simulink model "sampleModel2087"  (R2023a)
settings: Solver=VariableStepAuto  StartTime=0.0  StopTime=10.0  RelTol=1e-3
libraries: simulink x4, hdlsllib x3
settings Model: Creator=user1  LastModifiedBy=user1

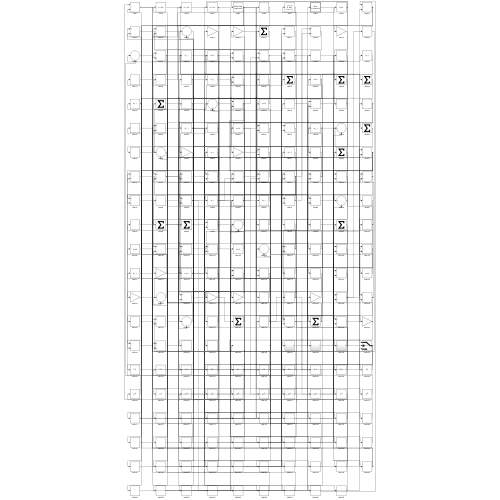
[thumbnail: Simulink's stored preview of the top-level diagram]
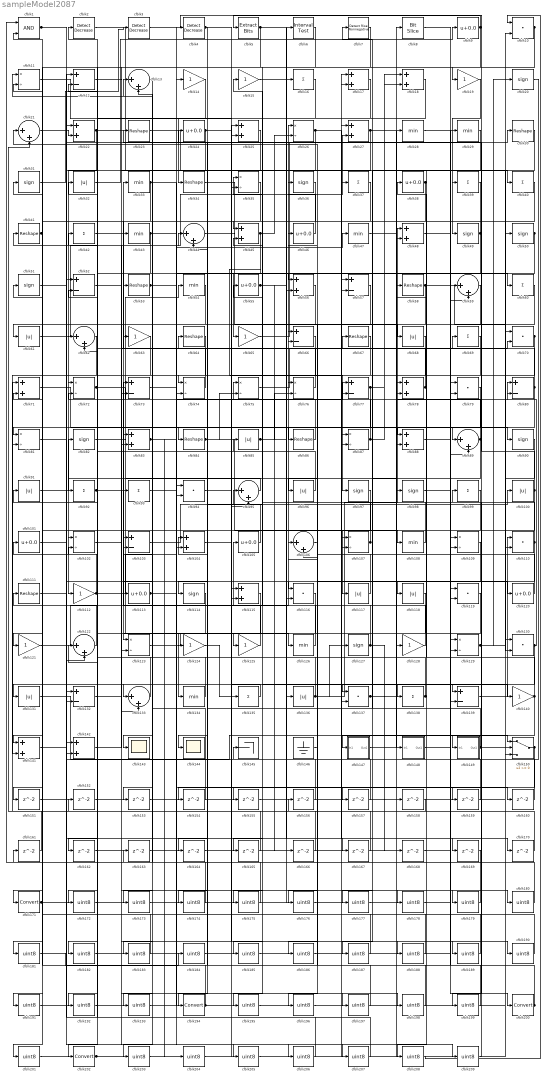
== system sampleModel2087 ==
  cfblk1 : Logic  AllPortsSameDT=off  OutDataTypeStr=boolean
  cfblk{10,70,79,94,110,116,119,130,137} (9 alike) : DotProduct  OutDataTypeStr=Inherit: Inherit via internal rule
  cfblk{32,61,68,85,91,96,100,117..118,131,136} (11 alike) : Abs  SaturateOnIntegerOverflow=off
  cfblk{9,24,38,46,55,101,105,113,120} (9 alike) : Bias  Bias=0.0  SaturateOnIntegerOverflow=off
  cfblk{11,26,35,72,74..76,81,87,102,107,109,123,129} (14 alike) : Product  Inputs=*/  RndMeth=Zero  SaturateOnIntegerOverflow=on
  cfblk{12,52,57,66,73,77,80,103,132,139} (10 alike) : Sum  Inputs=+-
  cfblk{17..18,22,25,27,45,48,56,71,78,83,88,104,115,141..142} (16 alike) : Sum
  cfblk{13,21,44,59,62,89,95,106,122,133} (10 alike) : Sum  Inputs=|++
  cfblk{28..29,33,43,47,54,108,126,134} (9 alike) : MinMax
  cfblk{23,30,34,41,53,58,64,67,84,86,111} (11 alike) : Reshape
  cfblk{14..15,19,63,65,112,121,124..125,128,140} (11 alike) : Gain
  cfblk{20,31,36,49..51,82,90,97..98,114,127} (12 alike) : Signum
  cfblk{16,37,39..40,42,60,69,92..93,99,135,138} (12 alike) : Sum  Inputs=+
  cfblk143 : Scope
  cfblk144 : Scope
  cfblk145 : Terminator
  cfblk146 : Ground
  cfblk147 : Subsystem
      settings: LibrarySourceBlock=|
      | hdlsllib/Ports &
      | Subsystems/Subsystem
  cfblk148 : Subsystem
      settings: LibrarySourceBlock=|
      | hdlsllib/Ports &
      | Subsystems/Subsystem
  cfblk149 : Subsystem
      settings: LibrarySourceBlock=|
      | hdlsllib/Ports &
      | Subsystems/Subsystem
  cfblk150 : Switch  SaturateOnIntegerOverflow=off  InputSameDT=off
  cfblk{151..170} (20 alike) : Delay  SampleTime=1
  cfblk{171,194,200,202} (4 alike) : DataTypeConversion  SaturateOnIntegerOverflow=off  RndMeth=Floor
  cfblk{172..193,195..199,201,203..209} (35 alike) : DataTypeConversion  OutDataTypeStr=uint8  SaturateOnIntegerOverflow=off  RndMeth=Floor
  cfblk2 : simulink/Logic and Bit Operations/Detect Decrease  vinit=0.0  OutDataTypeStr=boolean
      settings: LibrarySourceBlock=|
      | hdlsllib/Logic and Bit
      | Operations/Detect
      | Decrease
  cfblk3 : simulink/Logic and Bit Operations/Detect Decrease  vinit=0.0  OutDataTypeStr=boolean
      settings: LibrarySourceBlock=|
      | hdlsllib/Logic and Bit
      | Operations/Detect
      | Decrease
  cfblk4 : simulink/Logic and Bit Operations/Detect Decrease  vinit=0.0  OutDataTypeStr=boolean
      settings: LibrarySourceBlock=|
      | hdlsllib/Logic and Bit
      | Operations/Detect
      | Decrease
  cfblk5 : simulink/Logic and Bit Operations/Extract Bits  bitsToExtract=Upper half  numBits=8  bitIdxRange=[0 7]  outScalingMode=Preserve fixed-point scaling
      settings: LibrarySourceBlock=|
      | hdlsllib/Logic and Bit
      | Operations/Extract Bits
  cfblk6 : hdlsllib/Logic and Bit Operations/Interval Test  IntervalClosedRight=on  uplimit=0.5  IntervalClosedLeft=on  lowlimit=-0.5  OutDataTypeStr=boolean
  cfblk7 : hdlsllib/Logic and Bit Operations/Detect Rise Nonnegative  vinit=0  OutDataTypeStr=boolean
  cfblk8 : hdlsllib/Logic and Bit Operations/Bit Slice  lidx=7  ridx=0
  wires:
  cfblk127/1 -> cfblk105/1, cfblk45/2, cfblk168/1
  cfblk50/1 -> cfblk65/1, cfblk143/1
  cfblk130/1 -> cfblk80/2, cfblk165/1
  cfblk110/1 -> cfblk54/1, cfblk147/1(In1), cfblk199/1
  cfblk42/1 -> cfblk125/1
  cfblk150/1 -> cfblk154/1, cfblk155/1
  cfblk125/1 -> cfblk73/1
  cfblk45/1 -> cfblk97/1, cfblk26/2, cfblk62/2
  cfblk56/1 -> cfblk61/1
  cfblk80/1 -> cfblk33/1, cfblk96/1
  cfblk103/1 -> cfblk100/1
  cfblk129/1 -> cfblk50/1, cfblk20/1
  cfblk22/1 -> cfblk112/1, cfblk57/1
  cfblk25/1 -> cfblk123/1
  cfblk91/1 -> cfblk82/1
  cfblk84/1 -> cfblk108/1, cfblk75/2, cfblk188/1
  cfblk29/1 -> cfblk118/1
  cfblk71/1 -> cfblk89/1
  cfblk72/1 -> cfblk134/1, cfblk102/1, cfblk133/2
  cfblk32/1 -> cfblk9/1
  cfblk139/1 -> cfblk110/1
  cfblk136/1 -> cfblk48/1, cfblk24/1, cfblk127/1
  cfblk20/1 -> cfblk145/1
  cfblk19/1 -> cfblk49/1
  cfblk92/1 -> cfblk44/1, cfblk190/1
  cfblk41/1 -> cfblk11/2, cfblk151/1
  cfblk16/1 -> cfblk133/1
  cfblk38/1 -> cfblk74/1, cfblk53/1
  cfblk142/1 -> cfblk93/1
  cfblk121/1 -> cfblk26/1
  cfblk43/1 -> cfblk63/1, cfblk57/2
  cfblk59/1 -> cfblk103/1
  cfblk100/1 -> cfblk117/1, cfblk23/1
  cfblk2/1 -> cfblk130/1
  cfblk65/1 -> cfblk8/1
  cfblk115/1 -> cfblk202/1
  cfblk131/1 -> cfblk149/1(In1)
  cfblk133/1 -> cfblk91/1
  cfblk31/1 -> cfblk3/1
  cfblk96/1 -> cfblk42/1
  cfblk46/1 -> cfblk36/1
  cfblk44/1 -> cfblk56/1
  cfblk82/1 -> cfblk148/1(In1)
  cfblk95/1 -> cfblk92/1
  cfblk87/1 -> cfblk66/1, cfblk18/2
  cfblk88/1 -> cfblk90/1
  cfblk128/1 -> cfblk85/1
  cfblk28/1 -> cfblk200/1
  cfblk53/1 -> cfblk88/1, cfblk116/1, cfblk207/1
  cfblk60/1 -> cfblk114/1
  cfblk11/1 -> cfblk25/2
  cfblk134/1 -> cfblk111/1
  cfblk33/1 -> cfblk191/1, cfblk198/1
  cfblk63/1 -> cfblk141/1
  cfblk3/1 -> cfblk19/1
  cfblk74/1 -> cfblk41/1
  cfblk75/1 -> cfblk69/1
  cfblk86/1 -> cfblk15/1
  cfblk140/1 -> cfblk58/1, cfblk177/1
  cfblk132/1 -> cfblk70/2
  cfblk93/1 -> cfblk47/1
  cfblk18/1 -> cfblk34/1
  cfblk17/1 -> cfblk194/1
  cfblk24/1 -> cfblk40/1, cfblk73/2
  cfblk124/1 -> cfblk135/1
  cfblk57/1 -> cfblk86/1
  cfblk146/1 -> cfblk76/1
  cfblk85/1 -> cfblk140/1, cfblk55/1, cfblk76/2
  cfblk5/1 -> cfblk121/1, cfblk88/2, cfblk123/2, cfblk60/1, cfblk62/1
  cfblk138/1 -> cfblk101/1, cfblk102/2
  cfblk55/1 -> cfblk16/1, cfblk166/1
  cfblk105/1 -> cfblk64/1
  cfblk40/1 -> cfblk43/1
  cfblk112/1 -> cfblk4/1, cfblk31/1
  cfblk126/1 -> cfblk95/1
  cfblk123/1 -> cfblk126/1
  cfblk34/1 -> cfblk68/1
  cfblk101/1 -> cfblk122/2
  cfblk70/1 -> cfblk138/1, cfblk79/2, cfblk175/1, cfblk196/1
  cfblk120/1 -> cfblk75/1
  cfblk62/1 -> cfblk141/2
  cfblk76/1 -> cfblk2/1
  cfblk117/1 -> cfblk21/1
  cfblk147/1(Out1) -> cfblk128/1
  cfblk90/1 -> cfblk110/2
  cfblk148/1(Out1) -> cfblk29/1
  cfblk141/1 -> cfblk30/1
  cfblk81/1 -> cfblk120/1
  cfblk122/1 -> cfblk71/2
  cfblk108/1 -> cfblk67/1
  cfblk89/1 -> cfblk32/1, cfblk137/1
  cfblk39/1 -> cfblk113/1
  cfblk135/1 -> cfblk131/1
  cfblk10/1 -> cfblk124/1, cfblk159/1
  cfblk107/1 -> cfblk46/1, cfblk72/2
  cfblk61/1 -> cfblk27/2
  cfblk58/1 -> cfblk130/2, cfblk83/2
  cfblk83/1 -> cfblk204/1, cfblk206/1
  cfblk113/1 -> cfblk77/1, cfblk178/1
  cfblk54/1 -> cfblk83/1
  cfblk21/1 -> cfblk22/2
  cfblk6/1 -> cfblk171/1
  cfblk27/1 -> cfblk139/1, cfblk153/1
  cfblk78/1 -> cfblk38/1, cfblk35/1
  cfblk26/1 -> cfblk116/2, cfblk169/1
  cfblk23/1 -> cfblk39/1
  cfblk66/1 -> cfblk81/1
  cfblk98/1 -> cfblk59/1
  cfblk64/1 -> cfblk72/1
  cfblk137/1 -> cfblk80/1, cfblk158/1
  cfblk48/1 -> cfblk129/1
  cfblk1/1 -> cfblk132/2, cfblk35/2
  cfblk77/1 -> cfblk84/1, cfblk81/2, cfblk18/1, cfblk182/1
  cfblk79/1 -> cfblk129/2
  cfblk67/1 -> cfblk87/2
  cfblk4/1 -> cfblk139/2, cfblk174/1
  cfblk8/1 -> cfblk150/1
  cfblk149/1(Out1) -> cfblk104/1, cfblk150/2, cfblk7/1
  cfblk9/1 -> cfblk142/2, cfblk5/1
  cfblk68/1 -> cfblk104/2
  cfblk47/1 -> cfblk98/1
  cfblk49/1 -> cfblk144/1, cfblk45/1
  cfblk151/1 -> cfblk78/1
  cfblk152/1 -> cfblk70/1
  cfblk153/1 -> cfblk74/2
  cfblk154/1 -> cfblk11/1
  cfblk155/1 -> cfblk56/2
  cfblk156/1 -> cfblk122/1
  cfblk73/1 -> cfblk157/1
  cfblk157/1 -> cfblk27/1
  cfblk158/1 -> cfblk21/2
  cfblk159/1 -> cfblk22/1
  cfblk104/1 -> cfblk160/1
  cfblk160/1 -> cfblk142/1
  cfblk161/1 -> cfblk71/1
  cfblk36/1 -> cfblk162/1
  cfblk162/1 -> cfblk95/2
  cfblk118/1 -> cfblk164/1
  cfblk164/1 -> cfblk89/2
  cfblk165/1 -> cfblk25/1
  cfblk166/1 -> cfblk1/2
  cfblk15/1 -> cfblk167/1
  cfblk167/1 -> cfblk103/2
  cfblk168/1 -> cfblk59/2
  cfblk169/1 -> cfblk1/1
  cfblk51/1 -> cfblk170/1
  cfblk170/1 -> cfblk66/2
  cfblk171/1 -> cfblk77/2, cfblk136/1
  cfblk35/1 -> cfblk172/1
  cfblk172/1 -> cfblk6/1
  cfblk13/1 -> cfblk173/1
  cfblk173/1 -> cfblk78/2
  cfblk174/1 -> cfblk13/1
  cfblk175/1 -> cfblk13/2
  cfblk109/1 -> cfblk176/1
  cfblk176/1 -> cfblk107/1
  cfblk177/1 -> cfblk109/1
  cfblk178/1 -> cfblk109/2
  cfblk163/1 -> cfblk179/1
  cfblk179/1 -> cfblk132/1
  cfblk102/1 -> cfblk180/1
  cfblk180/1 -> cfblk163/1
  cfblk37/1 -> cfblk181/1
  cfblk182/1 -> cfblk37/1
  cfblk119/1 -> cfblk183/1
  cfblk183/1 -> cfblk161/1
  cfblk181/1 -> cfblk184/1
  cfblk184/1 -> cfblk119/1
  cfblk7/1 -> cfblk185/1
  cfblk185/1 -> cfblk119/2
  cfblk106/1 -> cfblk186/1
  cfblk186/1 -> cfblk107/2
  cfblk30/1 -> cfblk187/1
  cfblk187/1 -> cfblk106/1
  cfblk188/1 -> cfblk106/2
  cfblk94/1 -> cfblk189/1
  cfblk189/1 -> cfblk152/1
  cfblk190/1 -> cfblk94/1
  cfblk191/1 -> cfblk94/2
  cfblk14/1 -> cfblk192/1
  cfblk192/1 -> cfblk87/1
  cfblk114/1 -> cfblk193/1
  cfblk193/1 -> cfblk14/1
  cfblk194/1 -> cfblk150/3, cfblk51/1
  cfblk69/1 -> cfblk195/1
  cfblk195/1 -> cfblk17/1
  cfblk196/1 -> cfblk17/2
  cfblk12/1 -> cfblk197/1
  cfblk197/1 -> cfblk156/1
  cfblk198/1 -> cfblk12/1
  cfblk199/1 -> cfblk12/2
  cfblk200/1 -> cfblk44/2, cfblk79/1
  cfblk97/1 -> cfblk201/1
  cfblk201/1 -> cfblk28/1
  cfblk202/1 -> cfblk137/2, cfblk48/2
  cfblk116/1 -> cfblk203/1
  cfblk203/1 -> cfblk115/1
  cfblk204/1 -> cfblk115/2
  cfblk52/1 -> cfblk205/1
  cfblk205/1 -> cfblk10/2
  cfblk206/1 -> cfblk52/1
  cfblk207/1 -> cfblk52/2
  cfblk99/1 -> cfblk208/1
  cfblk208/1 -> cfblk10/1
  cfblk111/1 -> cfblk209/1
  cfblk209/1 -> cfblk99/1

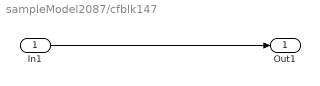
== system sampleModel2087/cfblk147 ==
  In1 : Inport
  Out1 : Outport
  wires:
  In1/1 -> Out1/1

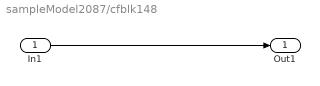
== system sampleModel2087/cfblk148 ==
  In1 : Inport
  Out1 : Outport
  wires:
  In1/1 -> Out1/1

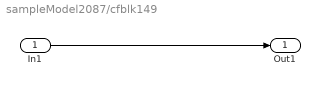
== system sampleModel2087/cfblk149 ==
  In1 : Inport
  Out1 : Outport
  wires:
  In1/1 -> Out1/1
